simulink model "lab1simu2"  (Simulink 7.7)
settings: Solver=ode45  StartTime=0.0  StopTime=10.0  RelTol=1e-3
settings Model: Creator=student  LastModifiedBy=mestan

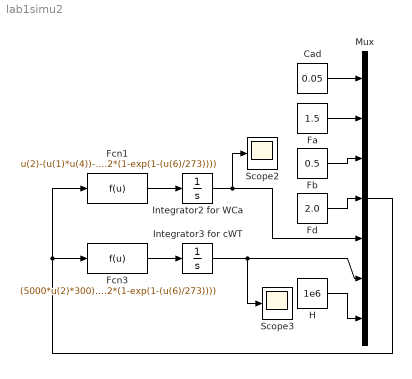
== system lab1simu2 ==
  Cad : Constant  Value=0.05
  Fa : Constant  Value=1.5
  Fb : Constant  Value=0.5
  Fcn1 : Fcn  Expr=u(2)-(u(1)*u(4))-(500*u(1)*0.2*(1-exp(1-(u(6)/273))))
  Fcn3 : Fcn  Expr=(5000*u(2)*300) + (5000*u(3)*300)-(5000*u(4)*400)+u(7)-(500*500*u(1)*0.2*(1-exp(1-(u(6)/273))))
  Fd : Constant  Value=2.0
  H : Constant  Value=1e6
  Integrator2 for WCa : Integrator  InitialCondition=1
  Integrator3 for cWT : Integrator  InitialCondition=300
  Mux : Mux  Inputs=7
  Scope2 : Scope
  Scope3 : Scope
      settings: SaveName=ScopeData2
  wires:
  Fa/1 -> Mux/2
  Fb/1 -> Mux/3
  Fd/1 -> Mux/4
  Mux/1 -> Fcn3/1, Fcn1/1
  Fcn1/1 -> Integrator2 for WCa/1
  Fcn3/1 -> Integrator3 for cWT/1
  Integrator2 for WCa/1 -> Mux/5, Scope2/1
  Integrator3 for cWT/1 -> Mux/6, Scope3/1
  H/1 -> Mux/7
  Cad/1 -> Mux/1
